simulink model "MotorControlLib"  (R2020b)
settings: Solver=VariableStepAuto  StartTime=0.0  StopTime=100  RelTol=1e-3
values from neighbouring files (symbols this model uses):
  Jm = 0.0000008    (= 8e-07)    [MotorControlLibData.m]    (also in local_pmsm_torque_control_data.m)
  Ld = 1.93E-5    [MotorControl.sldd]    (also in MotorControlLibData.m = 1.93e-05; local_pmsm_torque_control_data.m = 1.93e-05)
  LPF_BETA = 0.1    [ADCRawToIab.sldd]
  p = 4.0    [MotorControl.sldd]    (also in MotorControlLibData.m = 4; local_pmsm_torque_control_data.m = 4)
  Rs = 0.022    [MotorControl.sldd]    (also in MotorControlLibData.m = 0.022; local_pmsm_torque_control_data.m = 0.022)
  Vnom = 12.0    [MotorControl.sldd]    (also in MotorControlLibData.m = 12; local_pmsm_torque_control_data.m = 12)
undefined symbols (not defined in the file or in its folder): DiscIntNeverNeededParam
libraries: mcbcontrolslib x5, pid_lib x4, simulink x3, mcbpositiondecoderlib x1, autolibpmsmexterior x1, eeDqVoltageLimiter x1
settings Model: DataDictionary=MotorControl.sldd  NumberOfSteps=36  Creator=unix  LastModifiedBy=unix

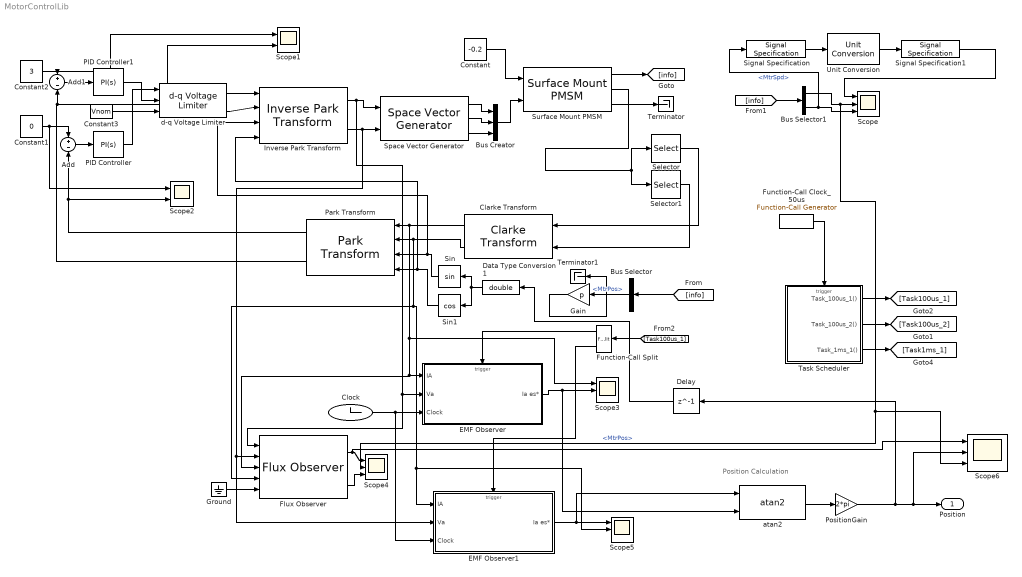
== system MotorControlLib ==
  note: Position Calculation
  Add : Sum  Inputs=+|-
  Add1 : Sum  Inputs=+|-
  Bus Creator : BusCreator  Inputs=3
  Bus Selector : BusSelector  OutputSignals=MtrPos
  Bus Selector1 : BusSelector  OutputSignals=MtrPos,MtrSpd
  Clarke Transform : mcbcontrolslib/Clarke Transform  VariantControl=Variant2
  Clock : Clock
  Constant : Constant  Value=-0.2
  Constant1 : Constant  Value=0
  Constant2 : Constant  Value=3
  Constant3 : Constant  Value=Vnom
  Data Type Conversion1 : DataTypeConversion  OutDataTypeStr=double
  Delay : Delay  DelayLength=1
  EMF Observer : Subsystem
  EMF Observer1 : Subsystem
  Flux Observer : mcbpositiondecoderlib/Flux Observer  BlockInputUnit=SI unit  PerUnitVoltage=13.86  PerUnitCurrent=19.3  PositionSelect=on  FluxSelect=on  TorqueSelect=off  PolePairs=4  StatorResistance=0.36  StatorDAxisInductance=0.2e-3  BlockSampleTime=50e-6  PositionUnit=Radians  PositionDatatype=single  FluxUnit=Weber  PerUnitFlux=0.1  FluxDatatype=single  TorqueUnit=Nm  PerUnitTorque=100  TorqueDatatype=single
      settings: SourceProductBaseCode=MT
  Function-Call Clock_50us : simulink/Ports & Subsystems/Function-Call Generator  sample_time=5e-5  numberOfIterations=1  DisallowWideOutput=off
  Function-Call Split : FunctionCallSplit  IconShape=distinctive  NumOutputPorts=2  OutputPortLayout=default
  Gain : Gain  Gain=p
  Ground : Ground
  Inverse Park Transform : mcbcontrolslib/Inverse Park Transform  AxisAlignment=D-axis
  PID Controller : pid_lib/PID Controller  Controller=PI  Form=Parallel  TimeDomain=Continuous-time  UseExternalTs=off  SampleTime=-1  IntegratorMethod=Forward Euler  FilterMethod=Forward Euler  ControllerParametersSource=internal  P=100  I=20  D=0  UseFilter=on  N=100  TunerSelectOption=Transfer Function Based (PID Tuner App)  InitialConditionSource=internal  InitialConditionForIntegrator=0  InitialConditionForFilter=0  DifferentiatorICPrevScaledInput=0  ExternalReset=none  TrackingMode=off  Kt=1  LimitOutput=on  SatLimitsSource=internal  UpperSaturationLimit=10  LowerSaturationLimit=-10  LinearizeAsGain=on  AntiWindupMode=none  Kb=1  POutMin=[]  POutMax=[]  IOutMin=[]  IOutMax=[]  DOutMin=[]  DOutMax=[]  NOutMin=[]  NOutMax=[]  SumOutMin=[]  SumOutMax=[]  SaturationOutMin=[]  SaturationOutMax=[]  PParamMin=[]  PParamMax=[]  IParamMin=[]  IParamMax=[]  DParamMin=[]  DParamMax=[]  NParamMin=[]  NParamMax=[]  KbParamMin=[]  KbParamMax=[]  KtParamMin=[]  KtParamMax=[]  KbOutMin=[]  KbOutMax=[]  KtOutMin=[]  KtOutMax=[]  IntegratorOutMin=[]  IntegratorOutMax=[]  FilterOutMin=[]  FilterOutMax=[]  SumI1OutMin=[]  SumI1OutMax=[]  SumI2OutMin=[]  SumI2OutMax=[]  SumI3OutMin=[]  SumI3OutMax=[]  SumI4OutMin=[]  SumI4OutMax=[]  SumDOutMin=[]  SumDOutMax=[]  DifferentiatorOutMin=[]  DifferentiatorOutMax=[]  FilterDiffOutCoefMin=[]  FilterDiffOutCoefMax=[]  ReciprocalOutMin=[]  ReciprocalOutMax=[]  SumDenOutMin=[]  SumDenOutMax=[]  SumNumOutMin=[]  SumNumOutMax=[]  DivideOutMin=[]  DivideOutMax=[]  UdiffTsProdOutMin=[]  UdiffTsProdOutMax=[]  NTsProdOutMin=[]  NTsProdOutMax=[]  UintegralTsProdOutMin=[]  UintegralTsProdOutMax=[]  UngainTsProdOutMin=[]  UngainTsProdOutMax=[]  IntegratorContinuousStateAttributes=''  IntegratorStateMustResolveToSignalObject=off  IntegratorRTWStateStorageClass=Auto  FilterContinuousStateAttributes=''  FilterStateMustResolveToSignalObject=off  FilterRTWStateStorageClass=Auto  ParallelPVariant=InternalParameters  IdealPVariant=Disabled  IVariant=InternalParameters  DVariant=Disabled  IntegratorVariant=Continuous  SatVariant=Enabled  AWVariant=Passthrough  PCopyVariant=Disabled  TRVariant=Disabled  FdbkBlocksVariant=Forward  IdealPFdbkVariant=Disabled  SatFdbkVariant=Disabled  DerivativeFilterVariant=Disabled  NVariant=Disabled  NCopyVariant=Disabled_SignalSpec  FilterICVariant=Disabled  IntegratorICVariant=InternalICs  ExternalResetVariant=Disabled  TRSumVariant=Passthrough  SumFdbkVariant=Disabled  SumVariant=Sum_PI  TsampFilterVariant=InternalTs  TsampNgainVariant=Passthrough  TsampIntegralVariant=Passthrough  ExternalSaturationOutDataTypeStr=Inherit: Same as second input
  PID Controller1 : pid_lib/PID Controller  Controller=PI  Form=Parallel  TimeDomain=Continuous-time  UseExternalTs=off  SampleTime=-1  IntegratorMethod=Forward Euler  FilterMethod=Forward Euler  ControllerParametersSource=internal  P=800  I=100  D=0  UseFilter=on  N=100  TunerSelectOption=Transfer Function Based (PID Tuner App)  InitialConditionSource=internal  InitialConditionForIntegrator=0  InitialConditionForFilter=0  DifferentiatorICPrevScaledInput=0  ExternalReset=none  TrackingMode=off  Kt=1  LimitOutput=off  SatLimitsSource=internal  UpperSaturationLimit=inf  LowerSaturationLimit=-inf  LinearizeAsGain=on  AntiWindupMode=none  Kb=1  POutMin=[]  POutMax=[]  IOutMin=[]  IOutMax=[]  DOutMin=[]  DOutMax=[]  NOutMin=[]  NOutMax=[]  SumOutMin=[]  SumOutMax=[]  SaturationOutMin=[]  SaturationOutMax=[]  PParamMin=[]  PParamMax=[]  IParamMin=[]  IParamMax=[]  DParamMin=[]  DParamMax=[]  NParamMin=[]  NParamMax=[]  KbParamMin=[]  KbParamMax=[]  KtParamMin=[]  KtParamMax=[]  KbOutMin=[]  KbOutMax=[]  KtOutMin=[]  KtOutMax=[]  IntegratorOutMin=[]  IntegratorOutMax=[]  FilterOutMin=[]  FilterOutMax=[]  SumI1OutMin=[]  SumI1OutMax=[]  SumI2OutMin=[]  SumI2OutMax=[]  SumI3OutMin=[]  SumI3OutMax=[]  SumI4OutMin=[]  SumI4OutMax=[]  SumDOutMin=[]  SumDOutMax=[]  DifferentiatorOutMin=[]  DifferentiatorOutMax=[]  FilterDiffOutCoefMin=[]  FilterDiffOutCoefMax=[]  ReciprocalOutMin=[]  ReciprocalOutMax=[]  SumDenOutMin=[]  SumDenOutMax=[]  SumNumOutMin=[]  SumNumOutMax=[]  DivideOutMin=[]  DivideOutMax=[]  UdiffTsProdOutMin=[]  UdiffTsProdOutMax=[]  NTsProdOutMin=[]  NTsProdOutMax=[]  UintegralTsProdOutMin=[]  UintegralTsProdOutMax=[]  UngainTsProdOutMin=[]  UngainTsProdOutMax=[]  IntegratorContinuousStateAttributes=''  IntegratorStateMustResolveToSignalObject=off  IntegratorRTWStateStorageClass=Auto  FilterContinuousStateAttributes=''  FilterStateMustResolveToSignalObject=off  FilterRTWStateStorageClass=Auto  ParallelPVariant=InternalParameters  IdealPVariant=Disabled  IVariant=InternalParameters  DVariant=Disabled  IntegratorVariant=Continuous  SatVariant=Disabled  AWVariant=Passthrough  PCopyVariant=Disabled  TRVariant=Disabled  FdbkBlocksVariant=Forward  IdealPFdbkVariant=Disabled  SatFdbkVariant=Disabled  DerivativeFilterVariant=Disabled  NVariant=Disabled  NCopyVariant=Disabled_SignalSpec  FilterICVariant=Disabled  IntegratorICVariant=InternalICs  ExternalResetVariant=Disabled  TRSumVariant=Passthrough  SumFdbkVariant=Disabled  SumVariant=Sum_PI  TsampFilterVariant=InternalTs  TsampNgainVariant=Passthrough  TsampIntegralVariant=Passthrough  ExternalSaturationOutDataTypeStr=Inherit: Same as second input
  Park Transform : mcbcontrolslib/Park Transform  AxisAlignment=D-axis
      settings: SourceProductBaseCode=MT
  PositionGain : Gain  Gain=2*pi  OutDataTypeStr=single  RndMeth=Simplest
  Scope{,3..6} (5 alike) : Scope  NumInputPorts=3
  Scope1 : Scope  NumInputPorts=2
  Scope2 : Scope  NumInputPorts=2
  Selector : Selector  InputPortWidth=3  IndexOptions=Index vector (dialog)  Indices=1  OutputSizes=1
  Selector1 : Selector  InputPortWidth=3  IndexOptions=Index vector (dialog)  Indices=2  OutputSizes=1
  Signal Specification : SignalSpecification  Unit=rad/s
  Signal Specification1 : SignalSpecification  Unit=rpm
  Sin : Trigonometry
  Sin1 : Trigonometry  Operator=cos
  Space Vector Generator : mcbcontrolslib/Space Vector Generator
      settings: SourceProductBaseCode=MT
  Surface Mount PMSM : autolibpmsmexterior/Surface Mount PMSM  port_config=Torque  sim_type=Continuous  Ts=0.001  P=p  Rs=Rs  Ldq_=Ld  KConstText=Back-emf constant (Ke):  lambda_pm=0.2205  Ke=cBackEMF_VKPRM  Kt=1.323  mechanical=[Jm, 4.924e-4, 0]  idq0=[0 0]  theta_init=0  omega_init=0  KConst=0.2205  lambda_pm_calc=0.0021651  RefBlkName='autolibpmsmexterior/Surface Mount PMSM'  aMode=5  Ldq="[0.0017      0.0017]"
      settings: SourceProductBaseCode=PW,MT,UV,VE,VP
  Task Scheduler : Stateflow chart  TreatAsAtomicUnit=on
  Terminator : Terminator
  Terminator1 : Terminator
  Unit Conversion : UnitConversion
  atan2 : mcbcontrolslib/atan2  outputUnit=PerUnit
      settings: SourceProductBaseCode=MT
  d-q Voltage Limiter : eeDqVoltageLimiter/d-q Voltage Limiter  AxisPrio=D-axis  Ts=-1
      settings: SourceProductBaseCode=PS
  Position : Outport
  wires:
  Constant/1 -> Surface Mount PMSM/1
  Selector1/1 -> Clarke Transform/2
  Selector/1 -> Clarke Transform/1
  Clarke Transform/1 -> Scope3/1, Flux Observer/3, EMF Observer/1(IA), Park Transform/1
  Clarke Transform/2 -> Flux Observer/4, EMF Observer1/1(IA), Scope5/2, Park Transform/2
  [info] -> Bus Selector/1
  Surface Mount PMSM/1 -> [info]
  Bus Selector/1 -> Gain/1  "<MtrPos>"
  Sin/1 -> Inverse Park Transform/3, Park Transform/3
  Sin1/1 -> Inverse Park Transform/4, Park Transform/4
  Park Transform/1 -> Add/2, Scope2/2
  Constant1/1 -> Scope2/1, Add/1
  Add/1 -> PID Controller/1
  Park Transform/2 -> Scope1/2, Add1/2
  Add1/1 -> PID Controller1/1
  Constant2/1 -> Scope1/1, Add1/1
  PID Controller1/1 -> d-q Voltage Limiter/2
  PID Controller/1 -> d-q Voltage Limiter/1
  Inverse Park Transform/1 -> Space Vector Generator/1, Flux Observer/1, EMF Observer/2(Va)
  Space Vector Generator/1 -> Bus Creator/1
  Space Vector Generator/2 -> Bus Creator/2
  Space Vector Generator/3 -> Bus Creator/3
  Bus Selector1/2 -> Signal Specification/1, Scope/3  "<MtrSpd>"
  [info] -> Bus Selector1/1
  Bus Selector1/1 -> Scope6/3, Scope4/2, Scope/2  "<MtrPos>"
  Surface Mount PMSM/3 -> Terminator/1
  d-q Voltage Limiter/1 -> Inverse Park Transform/1
  d-q Voltage Limiter/2 -> Inverse Park Transform/2
  Constant3/1 -> d-q Voltage Limiter/3
  Signal Specification1/1 -> Scope/1
  Signal Specification/1 -> Unit Conversion/1
  Unit Conversion/1 -> Signal Specification1/1
  Task Scheduler/1(Task_100us_1()) -> [Task100us_1]
  Function-Call Clock_50us/1 -> Task Scheduler/Trigger
  Task Scheduler/3(Task_1ms_1()) -> [Task1ms_1]
  Task Scheduler/2(Task_100us_2()) -> [Task100us_2]
  Clock/1 -> EMF Observer1/3(Clock), EMF Observer/3(Clock)
  Ground/1 -> Flux Observer/5
  Flux Observer/2 -> Scope4/3
  Flux Observer/1 -> Scope6/1, Scope4/1
  Inverse Park Transform/2 -> EMF Observer1/2(Va), Flux Observer/2, Space Vector Generator/2
  [Task100us_1] -> Function-Call Split/1
  Function-Call Split/1 -> EMF Observer/Trigger
  Function-Call Split/2 -> EMF Observer1/Trigger
  EMF Observer/1(Ia es*) -> atan2/2, Scope3/2
  atan2/1 -> PositionGain/1
  EMF Observer1/1(Ia es*) -> atan2/1, Scope5/1
  PositionGain/1 -> Delay/1, Scope6/2, Position/1
  Gain/1 -> Terminator1/1
  Bus Creator/1 -> Surface Mount PMSM/2
  Surface Mount PMSM/2 -> Selector1/1, Selector/1
  Data Type Conversion1/1 -> Sin/1, Sin1/1
  Delay/1 -> Data Type Conversion1/1

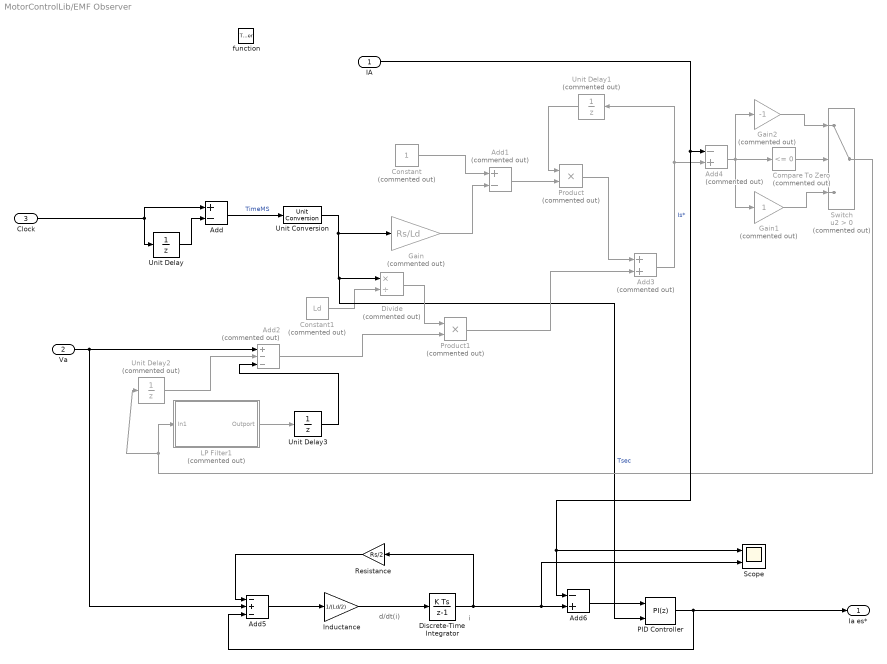
== system MotorControlLib/EMF Observer ==
  note: d/dt(i)
  note: i
  IA : Inport
  Va : Inport  Port=2
  Clock : Inport  Port=3
  function : TriggerPort  TriggerType=function-call  VariantControl=Variant
  Add : Sum  Inputs=+-
  Add1 : Sum  Commented=on  Inputs=+-
  Add2 : Sum  Commented=on  Inputs=+--
  Add3 : Sum  Commented=on
  Add4 : Sum  Commented=on  Inputs=-+
  Add5 : Sum  Inputs=-+-
  Add6 : Sum  Inputs=-+
  Compare To Zero : simulink/Logic and Bit Operations/Compare To Zero  Commented=on  relop=<=  OutDataTypeStr=boolean
  Constant : Constant  Commented=on  OutMin=0  OutMax=1  OutDataTypeStr=fixdt(0,8,2^-6,0)
  Constant1 : Constant  Commented=on  Value=Ld  OutMin=0  OutMax=1
  Discrete-Time Integrator : DiscreteIntegrator  gainval=1  SampleTime=-1  OutDataTypeStr=fixdt(1,32,2^-12,0)  UpperSaturationLimit=18  LowerSaturationLimit=-18  ICPrevOutput=DiscIntNeverNeededParam  ICPrevScaledInput=DiscIntNeverNeededParam
  Divide : Product  Commented=on  Inputs=*/
  Gain : Gain  Commented=on  Gain=Rs/Ld  OutDataTypeStr=fixdt(1,16,2^-8,0)
  Gain1 : Gain  Commented=on  OutDataTypeStr=Inherit: Inherit via back propagation
  Gain2 : Gain  Commented=on  Gain=-1
  Inductance : Gain  Gain=1/(Ld/2)
  LP Filter1 : Subsystem  Commented=on
  PID Controller : pid_lib/PID Controller  Controller=PI  Form=Parallel  TimeDomain=Discrete-time  UseExternalTs=on  SampleTime=-1  IntegratorMethod=Forward Euler  FilterMethod=Forward Euler  ControllerParametersSource=internal  P=0.11  I=1020  D=0  UseFilter=on  N=100  TunerSelectOption=Transfer Function Based (PID Tuner App)  InitialConditionSource=internal  InitialConditionForIntegrator=0  InitialConditionForFilter=0  DifferentiatorICPrevScaledInput=0  ExternalReset=none  TrackingMode=off  Kt=1  LimitOutput=off  SatLimitsSource=internal  UpperSaturationLimit=inf  LowerSaturationLimit=-inf  LinearizeAsGain=on  AntiWindupMode=none  Kb=1  POutMin=[]  POutMax=[]  IOutMin=[]  IOutMax=[]  DOutMin=[]  DOutMax=[]  NOutMin=[]  NOutMax=[]  SumOutMin=[]  SumOutMax=[]  SaturationOutMin=[]  SaturationOutMax=[]  PParamMin=[]  PParamMax=[]  IParamMin=[]  IParamMax=[]  DParamMin=[]  DParamMax=[]  NParamMin=[]  NParamMax=[]  KbParamMin=[]  KbParamMax=[]  KtParamMin=[]  KtParamMax=[]  KbOutMin=[]  KbOutMax=[]  KtOutMin=[]  KtOutMax=[]  IntegratorOutMin=[]  IntegratorOutMax=[]  FilterOutMin=[]  FilterOutMax=[]  SumI1OutMin=[]  SumI1OutMax=[]  SumI2OutMin=[]  SumI2OutMax=[]  SumI3OutMin=[]  SumI3OutMax=[]  SumI4OutMin=[]  SumI4OutMax=[]  SumDOutMin=[]  SumDOutMax=[]  DifferentiatorOutMin=[]  DifferentiatorOutMax=[]  FilterDiffOutCoefMin=[]  FilterDiffOutCoefMax=[]  ReciprocalOutMin=[]  ReciprocalOutMax=[]  SumDenOutMin=[]  SumDenOutMax=[]  SumNumOutMin=[]  SumNumOutMax=[]  DivideOutMin=[]  DivideOutMax=[]  UdiffTsProdOutMin=[]  UdiffTsProdOutMax=[]  NTsProdOutMin=[]  NTsProdOutMax=[]  UintegralTsProdOutMin=[]  UintegralTsProdOutMax=[]  UngainTsProdOutMin=[]  UngainTsProdOutMax=[]  IntegratorContinuousStateAttributes=''  IntegratorStateMustResolveToSignalObject=off  IntegratorRTWStateStorageClass=Auto  FilterContinuousStateAttributes=''  FilterStateMustResolveToSignalObject=off  FilterRTWStateStorageClass=Auto  ParallelPVariant=InternalParameters  IdealPVariant=Disabled  IVariant=InternalParameters  DVariant=Disabled  IntegratorVariant=Discrete  SatVariant=Disabled  AWVariant=Passthrough  PCopyVariant=Disabled  TRVariant=Disabled  FdbkBlocksVariant=Forward  IdealPFdbkVariant=Disabled  SatFdbkVariant=Disabled  DerivativeFilterVariant=Disabled  NVariant=Disabled  NCopyVariant=Disabled_SignalSpec  FilterICVariant=Disabled  IntegratorICVariant=InternalICs  ExternalResetVariant=Disabled  TRSumVariant=Passthrough  SumFdbkVariant=Disabled  SumVariant=Sum_PI  TsampFilterVariant=InternalTs  TsampNgainVariant=Passthrough  TsampIntegralVariant=ExternalTs  ExternalSaturationOutDataTypeStr=Inherit: Same as second input
  Product : Product  Commented=on
  Product1 : Product  Commented=on
  Resistance : Gain  Gain=Rs/2
  Scope : Scope  NumInputPorts=2
  Switch : Switch  Commented=on  Criteria=u2 > Threshold  OutDataTypeStr=fixdt(1,16,2^-9,0)
  Unit Conversion : UnitConversion  OutputType=Inherit: Inherit via back propagation
  Unit Delay : UnitDelay  SampleTime=-1  HasFrameUpgradeWarning=on
  Unit Delay1 : UnitDelay  Commented=on  SampleTime=-1  HasFrameUpgradeWarning=on
  Unit Delay2 : UnitDelay  Commented=on  SampleTime=-1  HasFrameUpgradeWarning=on
  Unit Delay3 : UnitDelay  SampleTime=-1  HasFrameUpgradeWarning=on
  Ia es* : Outport
  wires:
  Add/1 -> Unit Conversion/1  "TimeMS"
  Unit Delay1/1 -> Product/1
  Add2/1 -> Product1/2
  LP Filter1/1(Outport) -> Unit Delay3/1
  Constant1/1 -> Divide/2
  Gain2/1 -> Switch/1
  Product/1 -> Add3/1
  Add4/1 -> Gain1/1, Gain2/1, Compare To Zero/1
  Add3/1 -> Add4/2, Unit Delay1/1  "Is*"
  Clock/1 -> Unit Delay/1, Add/1
  Unit Delay2/1 -> Add2/2
  Add1/1 -> Product/2
  Compare To Zero/1 -> Switch/2
  Gain/1 -> Add1/2
  Unit Delay3/1 -> Add2/3
  Gain1/1 -> Switch/3
  Unit Conversion/1 -> Gain/1, PID Controller/2, Divide/1  "Tsec"
  Product1/1 -> Add3/2
  Switch/1 -> LP Filter1/1(In1), Unit Delay2/1
  Constant/1 -> Add1/1
  IA/1 -> Add6/1, Scope/1, Add4/1
  Unit Delay/1 -> Add/2
  Divide/1 -> Product1/1
  Resistance/1 -> Add5/1
  Add5/1 -> Inductance/1
  Va/1 -> Add5/2, Add2/1
  Inductance/1 -> Discrete-Time Integrator/1
  Discrete-Time Integrator/1 -> Scope/2, Add6/2, Resistance/1
  Add6/1 -> PID Controller/1
  PID Controller/1 -> Add5/3, Ia es*/1

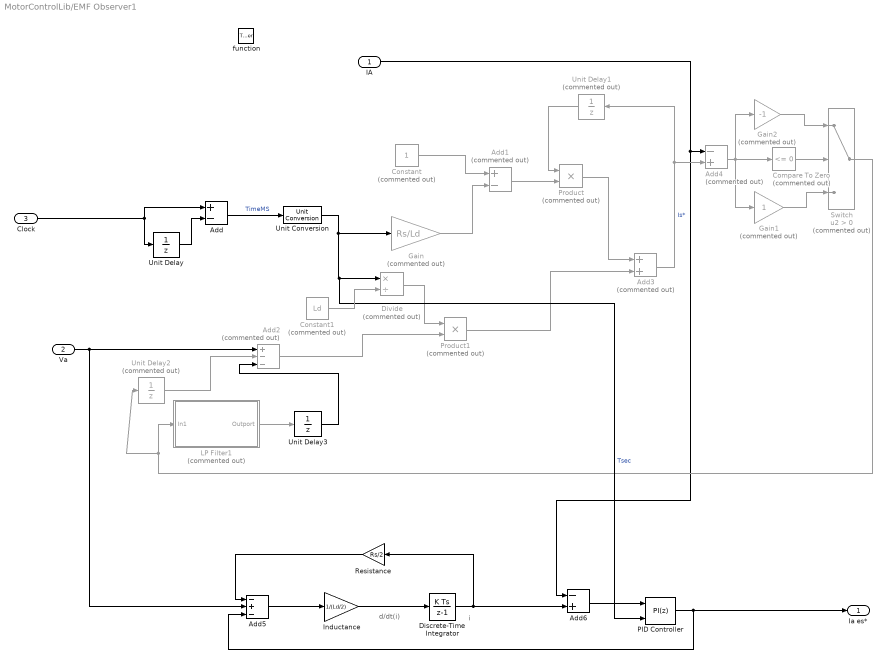
== system MotorControlLib/EMF Observer1 ==
  note: i
  note: d/dt(i)
  IA : Inport
  Va : Inport  Port=2
  Clock : Inport  Port=3
  function : TriggerPort  TriggerType=function-call  VariantControl=Variant
  Add : Sum  Inputs=+-
  Add1 : Sum  Commented=on  Inputs=+-
  Add2 : Sum  Commented=on  Inputs=+--
  Add3 : Sum  Commented=on
  Add4 : Sum  Commented=on  Inputs=-+
  Add5 : Sum  Inputs=-+-
  Add6 : Sum  Inputs=-+
  Compare To Zero : simulink/Logic and Bit Operations/Compare To Zero  Commented=on  relop=<=  OutDataTypeStr=boolean
  Constant : Constant  Commented=on  OutMin=0  OutMax=1  OutDataTypeStr=fixdt(0,8,2^-6,0)
  Constant1 : Constant  Commented=on  Value=Ld  OutMin=0  OutMax=1
  Discrete-Time Integrator : DiscreteIntegrator  gainval=1  SampleTime=-1  OutDataTypeStr=fixdt(1,32,2^-12,0)  UpperSaturationLimit=18  LowerSaturationLimit=-18  ICPrevOutput=DiscIntNeverNeededParam  ICPrevScaledInput=DiscIntNeverNeededParam
  Divide : Product  Commented=on  Inputs=*/
  Gain : Gain  Commented=on  Gain=Rs/Ld  OutDataTypeStr=fixdt(1,16,2^-8,0)
  Gain1 : Gain  Commented=on  OutDataTypeStr=Inherit: Inherit via back propagation
  Gain2 : Gain  Commented=on  Gain=-1
  Inductance : Gain  Gain=1/(Ld/2)
  LP Filter1 : Subsystem  Commented=on
  PID Controller : pid_lib/PID Controller  Controller=PI  Form=Parallel  TimeDomain=Discrete-time  UseExternalTs=on  SampleTime=-1  IntegratorMethod=Forward Euler  FilterMethod=Forward Euler  ControllerParametersSource=internal  P=0.11  I=1020  D=0  UseFilter=on  N=100  TunerSelectOption=Transfer Function Based (PID Tuner App)  InitialConditionSource=internal  InitialConditionForIntegrator=0  InitialConditionForFilter=0  DifferentiatorICPrevScaledInput=0  ExternalReset=none  TrackingMode=off  Kt=1  LimitOutput=off  SatLimitsSource=internal  UpperSaturationLimit=inf  LowerSaturationLimit=-inf  LinearizeAsGain=on  AntiWindupMode=none  Kb=1  POutMin=[]  POutMax=[]  IOutMin=[]  IOutMax=[]  DOutMin=[]  DOutMax=[]  NOutMin=[]  NOutMax=[]  SumOutMin=[]  SumOutMax=[]  SaturationOutMin=[]  SaturationOutMax=[]  PParamMin=[]  PParamMax=[]  IParamMin=[]  IParamMax=[]  DParamMin=[]  DParamMax=[]  NParamMin=[]  NParamMax=[]  KbParamMin=[]  KbParamMax=[]  KtParamMin=[]  KtParamMax=[]  KbOutMin=[]  KbOutMax=[]  KtOutMin=[]  KtOutMax=[]  IntegratorOutMin=[]  IntegratorOutMax=[]  FilterOutMin=[]  FilterOutMax=[]  SumI1OutMin=[]  SumI1OutMax=[]  SumI2OutMin=[]  SumI2OutMax=[]  SumI3OutMin=[]  SumI3OutMax=[]  SumI4OutMin=[]  SumI4OutMax=[]  SumDOutMin=[]  SumDOutMax=[]  DifferentiatorOutMin=[]  DifferentiatorOutMax=[]  FilterDiffOutCoefMin=[]  FilterDiffOutCoefMax=[]  ReciprocalOutMin=[]  ReciprocalOutMax=[]  SumDenOutMin=[]  SumDenOutMax=[]  SumNumOutMin=[]  SumNumOutMax=[]  DivideOutMin=[]  DivideOutMax=[]  UdiffTsProdOutMin=[]  UdiffTsProdOutMax=[]  NTsProdOutMin=[]  NTsProdOutMax=[]  UintegralTsProdOutMin=[]  UintegralTsProdOutMax=[]  UngainTsProdOutMin=[]  UngainTsProdOutMax=[]  IntegratorContinuousStateAttributes=''  IntegratorStateMustResolveToSignalObject=off  IntegratorRTWStateStorageClass=Auto  FilterContinuousStateAttributes=''  FilterStateMustResolveToSignalObject=off  FilterRTWStateStorageClass=Auto  ParallelPVariant=InternalParameters  IdealPVariant=Disabled  IVariant=InternalParameters  DVariant=Disabled  IntegratorVariant=Discrete  SatVariant=Disabled  AWVariant=Passthrough  PCopyVariant=Disabled  TRVariant=Disabled  FdbkBlocksVariant=Forward  IdealPFdbkVariant=Disabled  SatFdbkVariant=Disabled  DerivativeFilterVariant=Disabled  NVariant=Disabled  NCopyVariant=Disabled_SignalSpec  FilterICVariant=Disabled  IntegratorICVariant=InternalICs  ExternalResetVariant=Disabled  TRSumVariant=Passthrough  SumFdbkVariant=Disabled  SumVariant=Sum_PI  TsampFilterVariant=InternalTs  TsampNgainVariant=Passthrough  TsampIntegralVariant=ExternalTs  ExternalSaturationOutDataTypeStr=Inherit: Same as second input
  Product : Product  Commented=on
  Product1 : Product  Commented=on
  Resistance : Gain  Gain=Rs/2
  Switch : Switch  Commented=on  Criteria=u2 > Threshold  OutDataTypeStr=fixdt(1,16,2^-9,0)
  Unit Conversion : UnitConversion  OutputType=Inherit: Inherit via back propagation
  Unit Delay : UnitDelay  SampleTime=-1  HasFrameUpgradeWarning=on
  Unit Delay1 : UnitDelay  Commented=on  SampleTime=-1  HasFrameUpgradeWarning=on
  Unit Delay2 : UnitDelay  Commented=on  SampleTime=-1  HasFrameUpgradeWarning=on
  Unit Delay3 : UnitDelay  SampleTime=-1  HasFrameUpgradeWarning=on
  Ia es* : Outport
  wires:
  PID Controller/1 -> Ia es*/1, Add5/3
  Add6/1 -> PID Controller/1
  Discrete-Time Integrator/1 -> Resistance/1, Add6/2
  Inductance/1 -> Discrete-Time Integrator/1
  Va/1 -> Add2/1, Add5/2
  Add5/1 -> Inductance/1
  Resistance/1 -> Add5/1
  Divide/1 -> Product1/1
  Unit Delay/1 -> Add/2
  IA/1 -> Add4/1, Add6/1
  Constant/1 -> Add1/1
  Switch/1 -> Unit Delay2/1, LP Filter1/1(In1)
  Product1/1 -> Add3/2
  Unit Conversion/1 -> Divide/1, PID Controller/2, Gain/1  "Tsec"
  Gain1/1 -> Switch/3
  Unit Delay3/1 -> Add2/3
  Gain/1 -> Add1/2
  Compare To Zero/1 -> Switch/2
  Add1/1 -> Product/2
  Unit Delay2/1 -> Add2/2
  Clock/1 -> Add/1, Unit Delay/1
  Add3/1 -> Unit Delay1/1, Add4/2  "Is*"
  Add4/1 -> Compare To Zero/1, Gain2/1, Gain1/1
  Product/1 -> Add3/1
  Gain2/1 -> Switch/1
  Constant1/1 -> Divide/2
  LP Filter1/1(Outport) -> Unit Delay3/1
  Add2/1 -> Product1/2
  Unit Delay1/1 -> Product/1
  Add/1 -> Unit Conversion/1  "TimeMS"

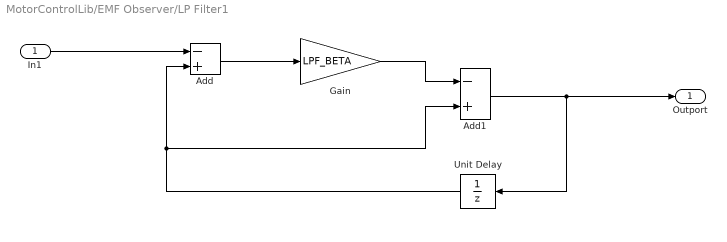
== system MotorControlLib/EMF Observer/LP Filter1 ==
  In1 : Inport
  Add : Sum  Inputs=-+
  Add1 : Sum  Inputs=-+
  Gain : Gain  Gain=LPF_BETA  OutDataTypeStr=Inherit: Inherit via back propagation
  Unit Delay : UnitDelay  SampleTime=-1  HasFrameUpgradeWarning=on
  Outport : Outport  OutDataTypeStr=fixdt(1,16,2^-8,0)
  wires:
  Gain/1 -> Add1/1
  In1/1 -> Add/1
  Add/1 -> Gain/1
  Unit Delay/1 -> Add1/2, Add/2
  Add1/1 -> Unit Delay/1, Outport/1

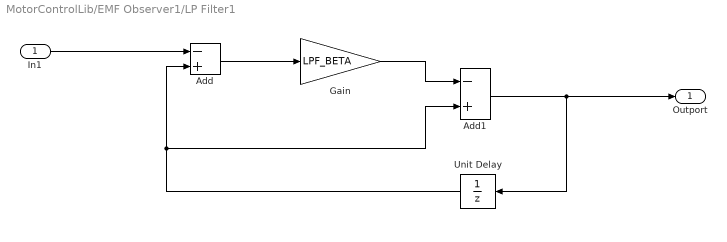
== system MotorControlLib/EMF Observer1/LP Filter1 ==
  In1 : Inport
  Add : Sum  Inputs=-+
  Add1 : Sum  Inputs=-+
  Gain : Gain  Gain=LPF_BETA  OutDataTypeStr=Inherit: Inherit via back propagation
  Unit Delay : UnitDelay  SampleTime=-1  HasFrameUpgradeWarning=on
  Outport : Outport  OutDataTypeStr=fixdt(1,16,2^-8,0)
  wires:
  Add1/1 -> Outport/1, Unit Delay/1
  Unit Delay/1 -> Add/2, Add1/2
  Add/1 -> Gain/1
  In1/1 -> Add/1
  Gain/1 -> Add1/1

== stateflow chart MotorControlLib/Task Scheduler ==
  (default) -> (junction 23) : CLK_50us
  (junction 23) -> (junction 17)
  (junction 17) -> (junction 22) [order 2]
  (junction 17) -> (junction 22) [order 1] : [cnt%%2==0]{Task_100us_1;}
  (junction 22) -> (junction 18) [order 2]
  (junction 22) -> (junction 18) [order 1] : [cnt%%2==0]{Task_100us_2;}
  (junction 18) -> (junction 21) [order 1] : [cnt%%20==0]{Task_1ms_1;}
  (junction 18) -> (junction 21) [order 2]
  (junction 21) -> (junction 34) [order 2]
  (junction 21) -> (junction 16) [order 1] : [1]{cnt++;}
  data: cnt local int32
  events: Task_100us_1 output FUNCTION_CALL_EVENT; Task_100us_2 output FUNCTION_CALL_EVENT; Task_1ms_1 output FUNCTION_CALL_EVENT; CLK_50us input FUNCTION_CALL_EVENT
